simulink model "Quadrotor_Model"  (R2016a)
settings: Solver=VariableStepAuto  StartTime=0.0  StopTime=20  RelTol=1e-3
settings Model: Creator=SRQ  LastModifiedBy=SRQ

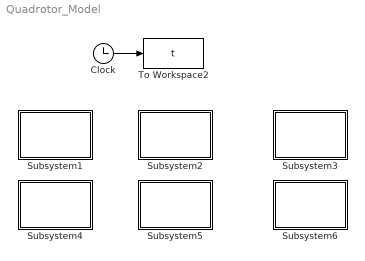
== system Quadrotor_Model ==
  Clock : Clock
  Subsystem1 : Subsystem
      mask Display: disp('俯仰通道');
  Subsystem2 : Subsystem
      mask Display: disp('翻滚通道');
  Subsystem3 : Subsystem
      mask Display: disp('偏航角');
  Subsystem4 : Subsystem
      mask Display: disp('X轴向与俯仰角');
  Subsystem5 : Subsystem
      mask Display: disp('Z轴');
  Subsystem6 : Subsystem
      mask Display: disp('Y轴向与翻滚角');
  To Workspace2 : ToWorkspace  VariableName=t  SampleTime=-1
  wires:
  Clock/1 -> To Workspace2/1

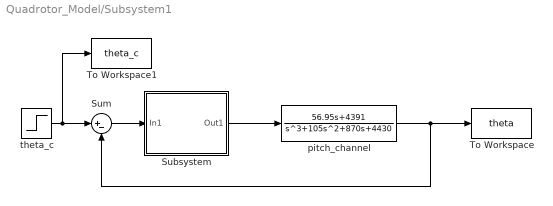
== system Quadrotor_Model/Subsystem1 ==
  Subsystem : Subsystem  mask{kp=1, ki=5, kd=0.01}
      mask Display: disp('PID');
  Sum : Sum  Inputs=|+-
  To Workspace : ToWorkspace  VariableName=theta  SampleTime=-1
  To Workspace1 : ToWorkspace  VariableName=theta_c  SampleTime=-1
  pitch_channel : TransferFcn  Numerator=[56.95 4391]  Denominator=[1 105 870 4430]
  theta_c : Step  Time=0  SampleTime=0
  wires:
  theta_c/1 -> To Workspace1/1, Sum/1
  Sum/1 -> Subsystem/1(In1)
  Subsystem/1(Out1) -> pitch_channel/1
  pitch_channel/1 -> Sum/2, To Workspace/1

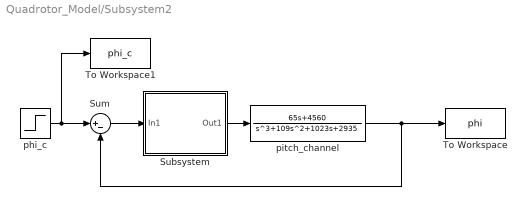
== system Quadrotor_Model/Subsystem2 ==
  Subsystem : Subsystem  mask{kp=2, ki=6, kd=0.1}
      mask Display: disp('PID');
  Sum : Sum  Inputs=|+-
  To Workspace : ToWorkspace  VariableName=phi  SampleTime=-1
  To Workspace1 : ToWorkspace  VariableName=phi_c  SampleTime=-1
  phi_c : Step  Time=0  SampleTime=0
  pitch_channel : TransferFcn  Numerator=[65 4560]  Denominator=[1 109 1023 2935]
  wires:
  phi_c/1 -> To Workspace1/1, Sum/1
  Sum/1 -> Subsystem/1(In1)
  Subsystem/1(Out1) -> pitch_channel/1
  pitch_channel/1 -> Sum/2, To Workspace/1

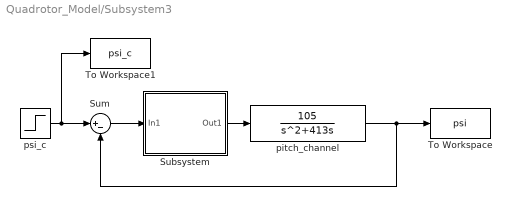
== system Quadrotor_Model/Subsystem3 ==
  Subsystem : Subsystem  mask{kp=3, ki=0.01, kd=1}
      mask Display: disp('PID');
  Sum : Sum  Inputs=|+-
  To Workspace : ToWorkspace  VariableName=psi  SampleTime=-1
  To Workspace1 : ToWorkspace  VariableName=psi_c  SampleTime=-1
  pitch_channel : TransferFcn  Numerator=[105]  Denominator=[1 413 0]
  psi_c : Step  Time=0  SampleTime=0
  wires:
  psi_c/1 -> To Workspace1/1, Sum/1
  Sum/1 -> Subsystem/1(In1)
  Subsystem/1(Out1) -> pitch_channel/1
  pitch_channel/1 -> Sum/2, To Workspace/1

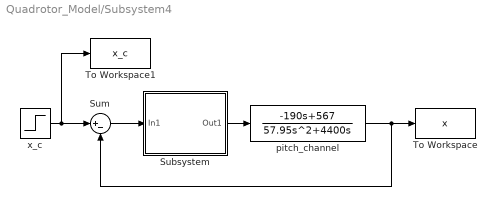
== system Quadrotor_Model/Subsystem4 ==
  Subsystem : Subsystem  mask{kp=10, ki=0.1, kd=0.1}
      mask Display: disp('PID');
  Sum : Sum  Inputs=|+-
  To Workspace : ToWorkspace  VariableName=x  SampleTime=-1
  To Workspace1 : ToWorkspace  VariableName=x_c  SampleTime=-1
  pitch_channel : TransferFcn  Numerator=[-190 567]  Denominator=[57.95 4400 0]
  x_c : Step  Time=0  SampleTime=0
  wires:
  x_c/1 -> To Workspace1/1, Sum/1
  Sum/1 -> Subsystem/1(In1)
  Subsystem/1(Out1) -> pitch_channel/1
  pitch_channel/1 -> Sum/2, To Workspace/1

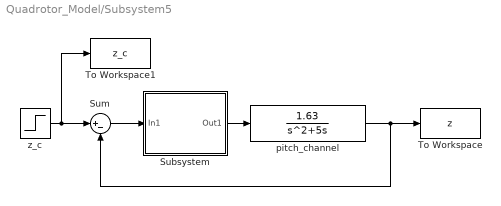
== system Quadrotor_Model/Subsystem5 ==
  Subsystem : Subsystem  mask{kp=3, ki=1, kd=1}
      mask Display: disp('PID');
  Sum : Sum  Inputs=|+-
  To Workspace : ToWorkspace  VariableName=z  SampleTime=-1
  To Workspace1 : ToWorkspace  VariableName=z_c  SampleTime=-1
  pitch_channel : TransferFcn  Numerator=[1.63]  Denominator=[1 5 0]
  z_c : Step  Time=0  SampleTime=0
  wires:
  z_c/1 -> To Workspace1/1, Sum/1
  Sum/1 -> Subsystem/1(In1)
  Subsystem/1(Out1) -> pitch_channel/1
  pitch_channel/1 -> Sum/2, To Workspace/1

== system Quadrotor_Model/Subsystem6 ==
  Subsystem : Subsystem  mask{kp=5, ki=0.01, kd=0.1}
      mask Display: disp('PID');
  Sum : Sum  Inputs=|+-
  To Workspace : ToWorkspace  VariableName=y  SampleTime=-1
  To Workspace1 : ToWorkspace  VariableName=y_c  SampleTime=-1
  pitch_channel : TransferFcn  Numerator=[-276.4 743.5]  Denominator=[61 4463 0]
  y_c : Step  Time=0  SampleTime=0
  wires:
  y_c/1 -> To Workspace1/1, Sum/1
  Sum/1 -> Subsystem/1(In1)
  Subsystem/1(Out1) -> pitch_channel/1
  pitch_channel/1 -> Sum/2, To Workspace/1

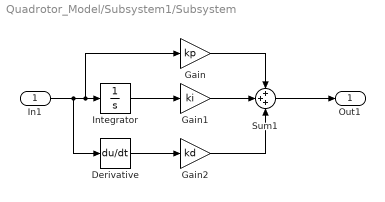
== system Quadrotor_Model/Subsystem1/Subsystem ==
  In1 : Inport
  Derivative : Derivative
  Gain : Gain  Gain=kp
  Gain1 : Gain  Gain=ki
  Gain2 : Gain  Gain=kd
  Integrator : Integrator
  Sum1 : Sum  Inputs=+++
  Out1 : Outport
  wires:
  Integrator/1 -> Gain1/1
  Derivative/1 -> Gain2/1
  Gain2/1 -> Sum1/3
  Gain/1 -> Sum1/1
  In1/1 -> Derivative/1, Gain/1, Integrator/1
  Sum1/1 -> Out1/1
  Gain1/1 -> Sum1/2

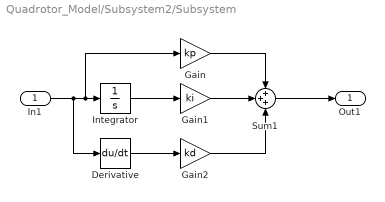
== system Quadrotor_Model/Subsystem2/Subsystem ==
  In1 : Inport
  Derivative : Derivative
  Gain : Gain  Gain=kp
  Gain1 : Gain  Gain=ki
  Gain2 : Gain  Gain=kd
  Integrator : Integrator
  Sum1 : Sum  Inputs=+++
  Out1 : Outport
  wires:
  Integrator/1 -> Gain1/1
  Derivative/1 -> Gain2/1
  Gain2/1 -> Sum1/3
  Gain/1 -> Sum1/1
  In1/1 -> Derivative/1, Gain/1, Integrator/1
  Sum1/1 -> Out1/1
  Gain1/1 -> Sum1/2

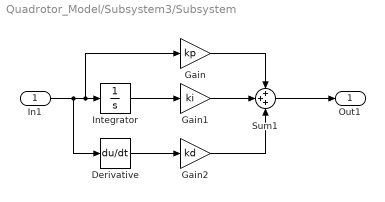
== system Quadrotor_Model/Subsystem3/Subsystem ==
  In1 : Inport
  Derivative : Derivative
  Gain : Gain  Gain=kp
  Gain1 : Gain  Gain=ki
  Gain2 : Gain  Gain=kd
  Integrator : Integrator
  Sum1 : Sum  Inputs=+++
  Out1 : Outport
  wires:
  Integrator/1 -> Gain1/1
  Derivative/1 -> Gain2/1
  Gain2/1 -> Sum1/3
  Gain/1 -> Sum1/1
  In1/1 -> Derivative/1, Gain/1, Integrator/1
  Sum1/1 -> Out1/1
  Gain1/1 -> Sum1/2

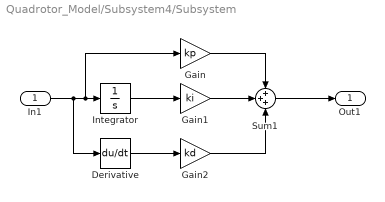
== system Quadrotor_Model/Subsystem4/Subsystem ==
  In1 : Inport
  Derivative : Derivative
  Gain : Gain  Gain=kp
  Gain1 : Gain  Gain=ki
  Gain2 : Gain  Gain=kd
  Integrator : Integrator
  Sum1 : Sum  Inputs=+++
  Out1 : Outport
  wires:
  Integrator/1 -> Gain1/1
  Derivative/1 -> Gain2/1
  Gain2/1 -> Sum1/3
  Gain/1 -> Sum1/1
  In1/1 -> Derivative/1, Gain/1, Integrator/1
  Sum1/1 -> Out1/1
  Gain1/1 -> Sum1/2

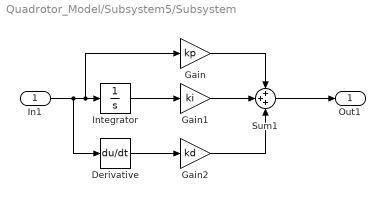
== system Quadrotor_Model/Subsystem5/Subsystem ==
  In1 : Inport
  Derivative : Derivative
  Gain : Gain  Gain=kp
  Gain1 : Gain  Gain=ki
  Gain2 : Gain  Gain=kd
  Integrator : Integrator
  Sum1 : Sum  Inputs=+++
  Out1 : Outport
  wires:
  Integrator/1 -> Gain1/1
  Derivative/1 -> Gain2/1
  Gain2/1 -> Sum1/3
  Gain/1 -> Sum1/1
  In1/1 -> Derivative/1, Gain/1, Integrator/1
  Sum1/1 -> Out1/1
  Gain1/1 -> Sum1/2

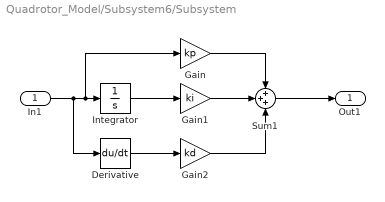
== system Quadrotor_Model/Subsystem6/Subsystem ==
  In1 : Inport
  Derivative : Derivative
  Gain : Gain  Gain=kp
  Gain1 : Gain  Gain=ki
  Gain2 : Gain  Gain=kd
  Integrator : Integrator
  Sum1 : Sum  Inputs=+++
  Out1 : Outport
  wires:
  Integrator/1 -> Gain1/1
  Derivative/1 -> Gain2/1
  Gain2/1 -> Sum1/3
  Gain/1 -> Sum1/1
  In1/1 -> Derivative/1, Gain/1, Integrator/1
  Sum1/1 -> Out1/1
  Gain1/1 -> Sum1/2
